simulink model "T37_SimulinkModelhw2_2021a"  (R2021a)
settings: Solver=ode4  StartTime=0.0  StopTime=10.0  RelTol=1e-3
undefined symbols (not defined in the file): Fax, Fay, Faz, Ftx, Fty, Ftz, g, Mx, My, Mz
libraries: simulink_extras x2, shared6dof x1
settings Model: OrderedModelArguments=off  Creator=Owner  LastModifiedBy=billy
settings DebuggingCC: UnconnectedInputMsg=none  UnconnectedOutputMsg=none  UnconnectedLineMsg=none  UnderSpecifiedDimensionMsg=warning
settings ModelReferenceCC: EnableRefExpFcnMdlSchedulingChecks=off
settings RTWCC: Description=Generic Real-Time Target  DLArmComputeVersion=20.02.1

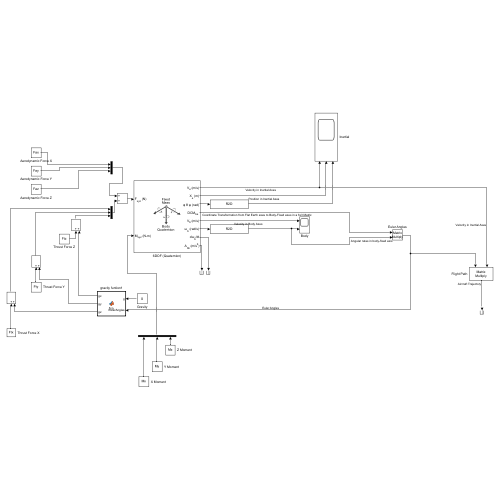
[thumbnail: Simulink's stored preview of the top-level diagram]
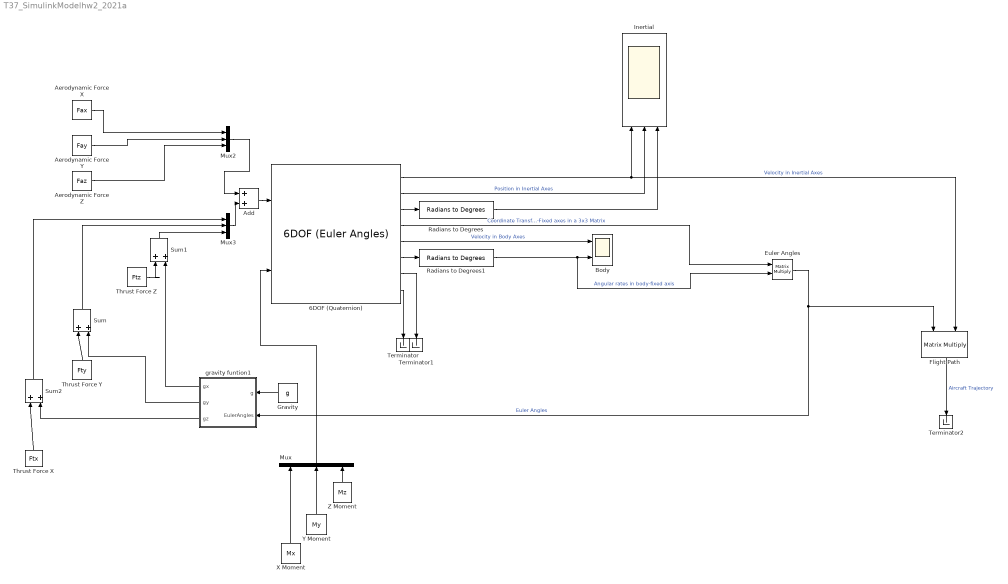
== system T37_SimulinkModelhw2_2021a ==
  6DOF (Quaternion) : shared6dof/6DOF (Euler Angles)  units=Metric (MKS)  mtype=Fixed  rep=Quaternion  xme_0=[0 0 0]  Vm_0=[0 0 0]  eul_0=[0 0 0]  pm_0=[0 0 0]  mass_0=1.0  mass_e=0.5  mass_f=2.0  inertia=eye(3)  inertia_e=eye(3)  inertia_f=2*eye(3)  k_quat=1.0  vre_flag=on  abi_flag=off  aMode=0  xme_statename=''  Vm_statename=''  eul_statename=''  quat_statename=''  pm_statename=''  mass_statename=''
  Add : Sum
  Aerodynamic Force X : Constant  Value=Fax
  Aerodynamic Force Y : Constant  Value=Fay
  Aerodynamic Force Z : Constant  Value=Faz
  Body : Scope  NumInputPorts=2
  Euler Angles : Product  Multiplication=Matrix(*)
  Flight Path : Product  Multiplication=Matrix(*)
  Gravity : Constant  Value=g
  Inertial : Scope  NumInputPorts=3
  Mux : Mux  Inputs=3
  Mux2 : Mux  Inputs=3
  Mux3 : Mux  Inputs=3
  Radians to Degrees : simulink_extras/Transformations/Radians to Degrees
  Radians to Degrees1 : simulink_extras/Transformations/Radians to Degrees
  Sum : Sum  Inputs=|++
  Sum1 : Sum  Inputs=|++
  Sum2 : Sum  Inputs=|++
  Terminator : Terminator
  Terminator1 : Terminator
  Terminator2 : Terminator
  Thrust Force X : Constant  Value=Ftx
  Thrust Force Y : Constant  Value=Fty
  Thrust Force Z : Constant  Value=Ftz
  X Moment : Constant  Value=Mx
  Y Moment : Constant  Value=My
  Z Moment : Constant  Value=Mz
  gravity funtion1 : MATLAB Function  TreatAsAtomicUnit=on
  wires:
  Aerodynamic Force Y/1 -> Mux2/2
  Aerodynamic Force X/1 -> Mux2/1
  Aerodynamic Force Z/1 -> Mux2/3
  Mux2/1 -> Add/1
  Mux3/1 -> Add/2
  Add/1 -> 6DOF (Quaternion)/1
  Mux/1 -> 6DOF (Quaternion)/2
  6DOF (Quaternion)/1 -> Flight Path/2, Inertial/1  "Velocity in Inertial Axes"
  6DOF (Quaternion)/2 -> Inertial/2  "Position in Inertial Axes"
  6DOF (Quaternion)/3 -> Radians to Degrees/1
  Radians to Degrees/1 -> Inertial/3
  6DOF (Quaternion)/4 -> Euler Angles/1  "Coordinate Transformation from Flat Earth axes to Body-Fixed axes in a 3x3 Matrix"
  6DOF (Quaternion)/8 -> Terminator/1
  6DOF (Quaternion)/7 -> Terminator1/1
  6DOF (Quaternion)/6 -> Radians to Degrees1/1
  6DOF (Quaternion)/5 -> Body/1  "Velocity in Body Axes"
  Radians to Degrees1/1 -> Euler Angles/2, Body/2  "Angular rates in body-fixed axis"
  Euler Angles/1 -> Flight Path/1, gravity funtion1/2(EulerAngles)  "Euler Angles"
  Gravity/1 -> gravity funtion1/1(g)
  gravity funtion1/1(gx) -> Sum1/2
  Thrust Force Z/1 -> Sum1/1
  Sum1/1 -> Mux3/3
  gravity funtion1/2(gy) -> Sum/2
  Thrust Force Y/1 -> Sum/1
  Sum/1 -> Mux3/2
  gravity funtion1/3(gz) -> Sum2/2
  Thrust Force X/1 -> Sum2/1
  Sum2/1 -> Mux3/1
  Z Moment/1 -> Mux/3
  Y Moment/1 -> Mux/2
  X Moment/1 -> Mux/1
  Flight Path/1 -> Terminator2/1  "Aircraft Trajectory"

== matlab function T37_SimulinkModelhw2_2021a/gravity funtion1 ==
  data: g input; gx output; gy output; gz output; EulerAngles input
function [gx, gy, gz] = fcn(g,EulerAngles)

gx = -g*sind(EulerAngles(2,1));
gy = g*((cosd(EulerAngles(2,1))).*(sind(EulerAngles(1,1))));
gz = g*((cosd(EulerAngles(2,1)).*(cosd(EulerAngles(1,1)))));


%function [gx, gy, gz] = fcn(g,phi, theta, psi)

%gx = -gsind(theta);
%gy = g*((cosd(theta)).*(sind(phi)));
%gz = g*((cosd(theta)).*(cosd(phi)));
